simulink model "Simulink_ass_III"  (R2024b)
settings: Solver=FixedStepAuto  StartTime=0.0  StopTime=inf  FixedStep=1/f_cmd  RelTol=1e-3
model workspace (MAT data in the model file):
  SL_ROS_VariableLengthArrays_MaxSizes.CommonInfo.ArrayTruncateAction = 'EmitWarning'
  SL_ROS_VariableLengthArrays_MaxSizes.MsgTypeMap = containers.Map
  SL_ROS_VariableLengthArrays_MaxSizes.MsgTypeMap.serialization.keys = {'sensor_msgs/Image'}
  SL_ROS_VariableLengthArrays_MaxSizes.MsgTypeMap.serialization.values{1}(1).PropertyName = 'Data'
  SL_ROS_VariableLengthArrays_MaxSizes.MsgTypeMap.serialization.values{1}(1).DataType = 'uint8'
  SL_ROS_VariableLengthArrays_MaxSizes.MsgTypeMap.serialization.values{1}(1).MaxLength = 921600
  SL_ROS_VariableLengthArrays_MaxSizes.MsgTypeMap.serialization.values{1}(2).PropertyName = 'Encoding'
  SL_ROS_VariableLengthArrays_MaxSizes.MsgTypeMap.serialization.values{1}(2).DataType = 'uint8'
  SL_ROS_VariableLengthArrays_MaxSizes.MsgTypeMap.serialization.values{1}(2).MaxLength = 128
  SL_ROS_VariableLengthArrays_MaxSizes.MsgTypeMap.serialization.uniformity = 0
  SL_ROS_VariableLengthArrays_MaxSizes.MsgTypeMap.serialization.keyType = 'char'
  SL_ROS_VariableLengthArrays_MaxSizes.MsgTypeMap.serialization.valueType = 'any'
values from neighbouring files (symbols this model uses):
  k_w = 1    [Assignment_III.m]
  max_vel = 0.2    [Assignment_III.m]
  yaw_rate_max = 0.4    [Assignment_III.m]
undefined symbols (not defined in the file or in its folder): Angular, Linear, Rec, SDTV
libraries: robotlib x9, simulink x6, visionstatistics x1, visionconversions x1
settings Model: Creator=vigno  LastModifiedBy=vigno
settings OptimizationCC: EnhancedBackFolding=on  PassReuseOutputArgsAs=Individual arguments  ZeroExternalMemoryAtStartup=off  ZeroInternalMemoryAtStartup=off  MaxStackSize=64  OptimizeBlockOrder=speed  DifferentSizesBufferReuse=on  OptimizationCustomize=off  EfficientTunableParamExpr=on
settings DebuggingCC: ParameterTunabilityLossMsg=error
settings HardwareCC: ProdBitPerPointer=32  ProdBitPerSizeT=32  ProdBitPerPtrDiffT=32  ProdLargestAtomicFloat=None  ProdIntDivRoundTo=Undefined  ProdEndianess=Unspecified  ProdWordSize=32  ProdHWDeviceType=Generic->Unspecified (assume 32-bit Generic)
settings ModelReferenceCC: EnableRefExpFcnMdlSchedulingChecks=on
settings SFSimCC: MATLABDynamicMemAlloc=off
settings RTWCC: Description=Embedded Coder  SystemTargetFile=ert.tlc  HardwareBoard=Robot Operating System (ROS)  TLCOptions="-aInlineSetEventsForThisBaseRateFcn=TLC_FALSE -aSuppressMultiTaskScheduler=TLC_FALSE  -aRateBasedStepFcn=0"  TemplateMakefile=ert_default_tmf  Toolchain=Catkin  TargetLang=C++  GPUComputeCapability=3.5
settings CodeAppCC: ForceParamTrailComments=on  IgnoreCustomStorageClasses=off  OperatorAnnotations=on  SimulinkDataObjDesc=on  SFDataObjDesc=on  InsertBlockDesc=on
settings ERTTargetCC: InlinedParameterPlacement=Hierarchical  DynamicArrayContainerType=coder::array

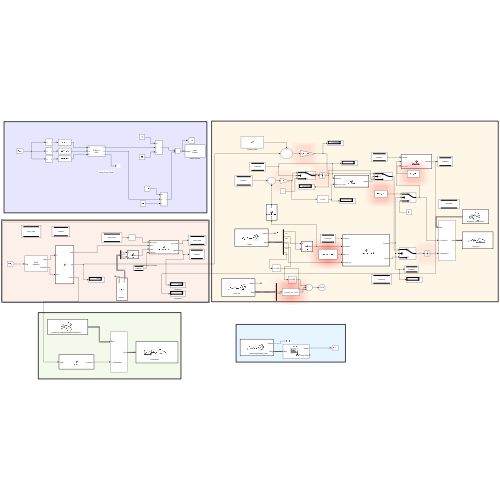
[thumbnail: Simulink's stored preview of the top-level diagram]
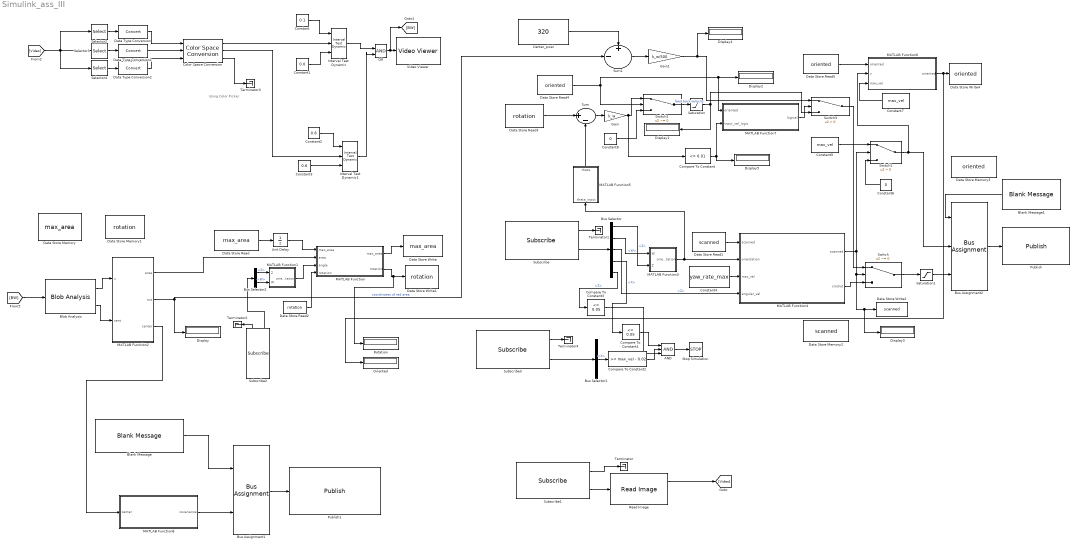
== system Simulink_ass_III ==
  note: Using Color Picker
  AND : Logic  Inputs=3  IconShape=distinctive  AllPortsSameDT=off  OutDataTypeStr=boolean
  Blank Message : robotlib/Blank Message  messageClass=Message  entityType=geometry_msgs/PoseWithCovariance  messageType=geometry_msgs/PoseWithCovariance  SampleTime=inf  legacyBusStruct=off
  Blank Message1 : robotlib/Blank Message  messageClass=Message  entityType=geometry_msgs/Twist  messageType=geometry_msgs/Twist  SampleTime=-1  legacyBusStruct=off
  Blob Analysis : visionstatistics/Blob Analysis  Tag=vipblks_row_conv  area=on  centroid=on  bBox=off  majorAxis=off  minorAxis=off  angle=off  eccentricity=off  equivDiameterSq=off  extent=off  perimeter=off  outDT=double  conn=8  isLabel=off  maxBlobs=5  warnIfNumBlobsExceeded=on  isCount=off  useMinArea=off  minArea=0  useMaxArea=off  maxArea=intmax('uint32')  excludeBorderBlob=off  isOutVarDim=off  isFill=on  fillValues=-1  roundingMode=Floor  overflowMode=off  prodOutputMode=Binary point scaling  prodOutputWordLength=32  prodOutputFracLength=16  accumMode=Binary point scaling  accumWordLength=32  accumFracLength=0  outputMode=Binary point scaling  outputWordLength=32  outputFracLength=16  firstCoeffMode=Binary point scaling  firstCoeffWordLength=16  firstCoeffFracLength=14  secondCoeffMode=Binary point scaling  secondCoeffWordLength=32  secondCoeffFracLength=16
  Bus Assignment1 : BusAssignment  AssignedSignals=Covariance
  Bus Assignment2 : BusAssignment  AssignedSignals=Linear.X,Angular.Z
  Bus Selector : BusSelector  OutputSignals=Pose.Pose.Orientation.Z,Pose.Pose.Orientation.W,Twist.Twist.Angular.Z,Twist.Twist.Linear.X,Twist.Twist.Angular.Z
  Bus Selector1 : BusSelector  OutputSignals=Linear.X
  Bus Selector2 : BusSelector  OutputSignals=Pose.Pose.Orientation.Z,Pose.Pose.Orientation.W
  Center_pixel : Constant  Value=320
  Color Space Conversion : visionconversions/Color Space  Conversion  conversion=Obsolete  conversionActive=R'G'B' to HSV  wp_str=D65  rec=Rec. 601 (SDTV)  sys=1125/60/2:1  imagePorts=Separate color signals
  Compare To Constant : simulink/Logic and Bit Operations/Compare To Constant  relop=<=  const=0.01  OutDataTypeStr=boolean
  Compare To Constant1 : simulink/Logic and Bit Operations/Compare To Constant  relop=<=  const=0.05  OutDataTypeStr=boolean
  Compare To Constant2 : simulink/Logic and Bit Operations/Compare To Constant  relop=>=  const=max_vel - 0.02  OutDataTypeStr=boolean
  Compare To Constant3 : simulink/Logic and Bit Operations/Compare To Constant  relop=<=  const=0.05  OutDataTypeStr=boolean
  Constant : Constant  Value=0.1
  Constant1 : Constant  Value=0.0
  Constant2 : Constant  Value=0.8
  Constant3 : Constant  Value=0.6
  Constant4 : Constant  Value=yaw_rate_max
  Constant5 : Constant  Value=max_vel
  Constant6 : Constant  Value=0
  Constant7 : Constant  Value=max_vel
  Constant8 : Constant  Value=0
  Data Store Memory : DataStoreMemory  DataStoreName=max_area  WriteAfterWriteMsg=warning  ShowAdditionalParam=off  OutDataTypeStr=int32
  Data Store Memory1 : DataStoreMemory  DataStoreName=rotation  WriteAfterWriteMsg=warning  ShowAdditionalParam=off
  Data Store Memory2 : DataStoreMemory  DataStoreName=scanned  WriteAfterWriteMsg=warning  ShowAdditionalParam=off  OutDataTypeStr=boolean
  Data Store Memory3 : DataStoreMemory  DataStoreName=oriented  WriteAfterWriteMsg=warning  ShowAdditionalParam=off  OutDataTypeStr=boolean
  Data Store Read : DataStoreRead  DataStoreName=max_area  DataStoreElements=max_area  IndexOptions=Index vector (dialog)  Indices=1  OutputSizes=1
  Data Store Read1 : DataStoreRead  DataStoreName=scanned  DataStoreElements=scanned  IndexOptions=Index vector (dialog)  Indices=1  OutputSizes=1
  Data Store Read2 : DataStoreRead  DataStoreName=rotation  IndexOptions=Index vector (dialog)  Indices=1  OutputSizes=1
  Data Store Read3 : DataStoreRead  DataStoreName=rotation  IndexOptions=Index vector (dialog)  Indices=1  OutputSizes=1
  Data Store Read4 : DataStoreRead  DataStoreName=oriented  IndexOptions=Index vector (dialog)  Indices=1  OutputSizes=1
  Data Store Read5 : DataStoreRead  DataStoreName=oriented  IndexOptions=Index vector (dialog)  Indices=1  OutputSizes=1
  Data Store Write : DataStoreWrite  DataStoreName=max_area  IndexOptions=Index vector (dialog)  Indices=1  OutputSizes=1
  Data Store Write1 : DataStoreWrite  DataStoreName=rotation  IndexOptions=Index vector (dialog)  Indices=1  OutputSizes=1
  Data Store Write2 : DataStoreWrite  DataStoreName=scanned  IndexOptions=Index vector (dialog)  Indices=1  OutputSizes=1
  Data Store Write4 : DataStoreWrite  DataStoreName=oriented  IndexOptions=Index vector (dialog)  Indices=1  OutputSizes=1
  Data Type Conversion : DataTypeConversion  SaturateOnIntegerOverflow=off  RndMeth=Floor
  Data Type Conversion1 : DataTypeConversion  SaturateOnIntegerOverflow=off  RndMeth=Floor
  Data Type Conversion2 : DataTypeConversion  SaturateOnIntegerOverflow=off  RndMeth=Floor
  Display{,1..5} (6 alike) : Display
  Gain : Gain  Gain=k_w
  Gain1 : Gain  Gain=k_w/500
  Interval Test Dynamic : simulink/Logic and Bit Operations/Interval Test Dynamic  IntervalClosedRight=on  IntervalClosedLeft=on  OutDataTypeStr=boolean
  Interval Test Dynamic1 : simulink/Logic and Bit Operations/Interval Test Dynamic  IntervalClosedRight=on  IntervalClosedLeft=on  OutDataTypeStr=boolean
  MATLAB Function : MATLAB Function  TreatAsAtomicUnit=on
  MATLAB Function1 : MATLAB Function  TreatAsAtomicUnit=on
  MATLAB Function2 : MATLAB Function  TreatAsAtomicUnit=on
  MATLAB Function3 : MATLAB Function  TreatAsAtomicUnit=on
  MATLAB Function4 : MATLAB Function  TreatAsAtomicUnit=on
  MATLAB Function5 : MATLAB Function  TreatAsAtomicUnit=on
  MATLAB Function6 : MATLAB Function  TreatAsAtomicUnit=on
  MATLAB Function7 : MATLAB Function  TreatAsAtomicUnit=on
  MATLAB Function8 : MATLAB Function  TreatAsAtomicUnit=on
  OR : Logic  IconShape=distinctive  AllPortsSameDT=off  OutDataTypeStr=boolean
  Oriented : Display
  Publish : robotlib/Publish  topicSource=Select from ROS network  topic=/cmd_vel  messageType=geometry_msgs/Twist  legacyBusStruct=off  messageQueueLength=1
  Publish1 : robotlib/Publish  topicSource=Specify your own  topic=/covariance  messageType=geometry_msgs/PoseWithCovariance  legacyBusStruct=off  messageQueueLength=1
  Read Image : robotlib/Read Image  MaximumImageSize=[480, 640]  ImageEncoding=rgb8  ShowAlphaOutput=off  ShowErrorCodeOutput=on  VariableSizeOutputs=off
  Rotation : Display
  Saturation : Saturate  UpperLimit=yaw_rate_max  LowerLimit=-yaw_rate_max
  Saturation1 : Saturate  UpperLimit=yaw_rate_max  LowerLimit=-yaw_rate_max
  Selector2 : Selector  NumberOfDimensions=3  InputPortWidth=3  IndexOptions=Index vector (dialog),Index vector (dialog),Index vector (dialog)  Indices=[1:480],[1:640],1  OutputSizes=1,1,1
  Selector3 : Selector  NumberOfDimensions=3  InputPortWidth=3  IndexOptions=Index vector (dialog),Index vector (dialog),Index vector (dialog)  Indices=[1:480],[1:640],2  OutputSizes=1,1,1
  Selector4 : Selector  NumberOfDimensions=3  InputPortWidth=3  IndexOptions=Index vector (dialog),Index vector (dialog),Index vector (dialog)  Indices=[1:480],[1:640],3  OutputSizes=1,1,1
  Stop Simulation : Stop
  Subscribe : robotlib/Subscribe  topicSource=Select from ROS network  topic=/odom  messageType=nav_msgs/Odometry  SampleTime=-1  legacyBusStruct=off  messageQueueLength=1
  Subscribe1 : robotlib/Subscribe  topicSource=Select from ROS network  topic=/camera/rgb/image_raw  messageType=sensor_msgs/Image  SampleTime=-1  legacyBusStruct=off  messageQueueLength=1
  Subscribe2 : robotlib/Subscribe  topicSource=Select from ROS network  topic=/odom  messageType=nav_msgs/Odometry  SampleTime=-1  legacyBusStruct=off  messageQueueLength=1
  Subscribe3 : robotlib/Subscribe  topicSource=Select from ROS network  topic=/cmd_vel  messageType=geometry_msgs/Twist  SampleTime=-1  legacyBusStruct=off  messageQueueLength=1
  Sum : Sum  Inputs=|+-
  Sum1 : Sum  Inputs=+-|
  Switch : Switch  Criteria=u2 ~= 0  SaturateOnIntegerOverflow=off  InputSameDT=off
  Switch1 : Switch  Criteria=u2 > Threshold  SaturateOnIntegerOverflow=off  InputSameDT=off
  Switch2 : Switch  Criteria=u2 ~= 0  SaturateOnIntegerOverflow=off  InputSameDT=off
  Switch3 : Switch  Criteria=u2 > Threshold  SaturateOnIntegerOverflow=off  InputSameDT=off
  Terminator{,1..4} (5 alike) : Terminator
  Unit Delay : UnitDelay  SampleTime=-1  HasFrameUpgradeWarning=on
  Video Viewer : VideoViewer  FigPos=[73 1078 1848 912]
  wires:
  Read Image/1 -> [Video]
  Subscribe1/2 -> Read Image/1
  Constant/1 -> Interval Test Dynamic/1
  [Video] -> Selector2/1, Selector3/1, Selector4/1
  Constant1/1 -> Interval Test Dynamic/3
  Blob Analysis/2 -> MATLAB Function2/2(cent)
  [BW] -> Blob Analysis/1
  MATLAB Function2/2(out) -> Display/1, Sum1/2  "coordinates of red area"
  Blob Analysis/1 -> MATLAB Function2/1(u)
  MATLAB Function/1(max_area) -> Data Store Write/1
  MATLAB Function/2(rotation) -> Rotation/1, Data Store Write1/1
  Subscribe1/1 -> Terminator/1
  Subscribe/1 -> Terminator1/1
  Subscribe2/1 -> Terminator2/1
  Bus Selector2/1 -> MATLAB Function1/1(Z)  "<Z>"
  Bus Selector2/2 -> MATLAB Function1/2(W)  "<W>"
  MATLAB Function1/1(orientation) -> MATLAB Function/3(angle)
  Subscribe2/2 -> Bus Selector2/1
  Subscribe/2 -> Bus Selector/1
  Bus Selector/1 -> MATLAB Function3/2(Z)  "<Z>"
  Bus Selector/2 -> MATLAB Function3/1(W)  "<W>"
  Blank Message1/1 -> Bus Assignment2/1
  Bus Assignment2/1 -> Publish/1
  Data Store Read1/1 -> MATLAB Function4/1("scanned ")
  Constant4/1 -> MATLAB Function4/3(max_vel)
  Bus Selector/3 -> MATLAB Function4/4(angular_vel)  "<Z>"
  Switch/1 -> Saturation1/1
  MATLAB Function4/1(scanned) -> Display3/1, Data Store Write2/1, Switch/2, Switch1/2
  MATLAB Function4/2(cmdrot) -> Switch/3
  Switch1/1 -> MATLAB Function6/2(v), Bus Assignment2/2
  Constant5/1 -> Switch1/1
  Constant6/1 -> Switch1/3
  Switch2/1 -> Saturation/1  "feed back velocity"
  Data Store Read2/1 -> MATLAB Function/4("rotation ")
  MATLAB Function3/1(orientation) -> MATLAB Function5/1(theta_input), MATLAB Function4/2(orientation)
  Data Store Read3/1 -> Sum/1
  Sum/1 -> Gain/1
  MATLAB Function6/1(oriented) -> Oriented/1, Data Store Write4/1
  Constant7/1 -> MATLAB Function6/3(max_vel)
  Data Store Read5/1 -> MATLAB Function6/1("oriented ")
  Center_pixel/1 -> Sum1/1
  Saturation/1 -> Switch3/3, Display1/1
  Sum1/1 -> Gain1/1
  Data Store Read4/1 -> Switch2/2, Display2/1, MATLAB Function7/1(oriented)
  MATLAB Function5/1(theta) -> Sum/2
  MATLAB Function2/1(area) -> MATLAB Function/2(area)
  Data Store Read/1 -> Unit Delay/1
  Unit Delay/1 -> MATLAB Function/1("max_area ")
  Selector2/1 -> Data Type Conversion/1
  Selector3/1 -> Data Type Conversion1/1
  Selector4/1 -> Data Type Conversion2/1
  Color Space Conversion/3 -> Terminator3/1
  Constant2/1 -> Interval Test Dynamic1/1
  Color Space Conversion/2 -> Interval Test Dynamic1/2
  Constant3/1 -> Interval Test Dynamic1/3
  Interval Test Dynamic1/1 -> OR/2
  OR/1 -> [BW], Video Viewer/1
  Data Type Conversion/1 -> Color Space Conversion/1
  Data Type Conversion2/1 -> Color Space Conversion/3
  Data Type Conversion1/1 -> Color Space Conversion/2
  Gain/1 -> Compare To Constant/1, Switch2/1
  Constant8/1 -> Switch2/3
  Gain1/1 -> Display4/1, Switch3/1
  Compare To Constant/1 -> Display5/1, MATLAB Function7/2(input_vel_logic)
  MATLAB Function7/1(logical) -> Switch3/2
  Switch3/1 -> Switch/1
  Subscribe3/1 -> Terminator4/1
  Subscribe3/2 -> Bus Selector1/1
  AND/1 -> Stop Simulation/1
  Bus Selector1/1 -> Compare To Constant2/1  "<X>"
  Compare To Constant2/1 -> AND/2
  Compare To Constant1/1 -> AND/1
  Bus Selector/4 -> Compare To Constant1/1  "<X>"
  Bus Selector/5 -> Compare To Constant3/1  "<Z>"
  Compare To Constant3/1 -> AND/3
  Interval Test Dynamic/1 -> OR/1
  Color Space Conversion/1 -> Interval Test Dynamic/2
  Blank Message/1 -> Bus Assignment1/1
  Bus Assignment1/1 -> Publish1/1
  MATLAB Function8/1(covariance) -> Bus Assignment1/2
  MATLAB Function2/3(center) -> MATLAB Function8/1(center)
  Saturation1/1 -> Bus Assignment2/3

== matlab function Simulink_ass_III/MATLAB Function3 ==
  data: W input; Z input; orientation output
function orientation = fcn(W, Z)
    orientation = 2 * atan2(Z, W);
    if orientation > pi
        orientation = orientation - 2 * pi;
    elseif orientation < -pi
        orientation = orientation + 2 * pi;
    end
end

== matlab function Simulink_ass_III/MATLAB Function ==
  data: max_area input; area input; max_area output; angle input; rotation output; rotation input
function [max_area, rotation] = findingRed(max_area, area, angle, rotation)    
    if area > max_area
        max_area = area;
        rotation = angle;
    end
end

== matlab function Simulink_ass_III/MATLAB Function2 ==
  data: area output; u input; cent input; out output; center output
function [area, out, center]  = fcn(u, cent)
    % Computers area of maximum area and the center
    [area, i] = max(u);
    out = cent(i, 1);
    if out == -1
        out = 320;
        center1 = 0;
    else
        center1 = out;
    end
    if cent(i, 2) == -1
        center2 = 0;
    else
        center2 = cent(i, 2);
    end
    center = [center1, center2];
end

== matlab function Simulink_ass_III/MATLAB Function4 ==
  data: scanned input; scanned output; orientation input; max_vel input; cmdrot output; angular_vel input
function [scanned, cmdrot] = scanEnvironment(scanned, orientation, max_vel, angular_vel)
    % Takes cmdrot and orientation as input, together with flag scanned: if
    % scanned is false, provides maximum velocity to the robot. If
    % orientation is null (starting position) but angular_vel is equal to
    % max_vel this means the robot has come back and scanned is true;
    % otherwise, it means that it has to go on.
    if ~ scanned
        if abs(angular_vel) < max_vel/4 
            cmdrot = max_vel/4;
        elseif abs(orientation) < 0.02
            scanned = true;
            cmdrot = 0;
        else
            cmdrot = max_vel;
        end
    else
        cmdrot = 0;
    end
end

== matlab function Simulink_ass_III/MATLAB Function1 ==
  data: Z input; orientation output; W input
function orientation = fcn(Z, W)
    orientation = 2 * atan2(Z, W);
    if orientation > pi
        orientation = orientation - 2 * pi;
    elseif orientation < -pi
        orientation = orientation + 2 * pi;
    end
end

== matlab function Simulink_ass_III/MATLAB Function5 ==
  data: theta_input input; theta output
function theta = correct_angle(theta_input)
    if theta_input <= pi && theta_input >= -pi
        theta = theta_input;
    else
        theta = mod(theta_input + pi, 2 * pi) - pi;
    end
end

== matlab function Simulink_ass_III/MATLAB Function6 ==
  data: oriented input; oriented output; v input; max_vel input
function oriented = allineator(oriented, v, max_vel)
    if v > (max_vel - 0.05) && oriented == false
        oriented = true;
    end
end

== matlab function Simulink_ass_III/MATLAB Function7 ==
  data: oriented input; logical output; input_vel_logic input
function logical = angular(oriented, input_vel_logic)
    % oriented and input_vel_logic: the latter indicates if orientation
    % difference is below a certain threshold. If so, selects the pixel
    % angular velocity.
    logical = 0;
    if oriented && input_vel_logic
        logical = 1;
    end
end

== matlab function Simulink_ass_III/MATLAB Function8 ==
  data: center input; covariance output
function covariance = juice(center)
    covariance = zeros(1, 36);
    covariance(1) = center(1);
    covariance(2) = center(2);
end
